simulink model "main_model"  (R2018b)
settings: Solver=VariableStepAuto  StartTime=0.0  StopTime=25  RelTol=1e-1
values from neighbouring files (symbols this model uses):
  beq = bm + bl/r^2    (= 1.5e-05)    [data.m]
  Cts = 1.091    [data.m]
  Jeq = Jm + Jl/r^2    (= 0.25041)    [data.m]
  lambda_rm = 0.01546    [data.m]
  Ld = 0.27e-3    (= 0.00027)    [data.m]
  Lls = 0.07e-3    (= 7e-05)    [data.m]
  Lq = 0.2e-3    (= 0.0002)    [data.m]
  Pp = 15    [data.m]
  r = 1    [data.m]
  Rs = 0.13    [data.m]
  Rts_amb = 55    [data.m]
  Tamb_max = 40    [data.m]
undefined symbols (not defined in the file or in its folder): ba, ke_omega, ke_theta, kei, ksa, ksia, R0p, Rdp, Rqp, sigbuilder_block
settings Model: Creator=Acer  LastModifiedBy=admin

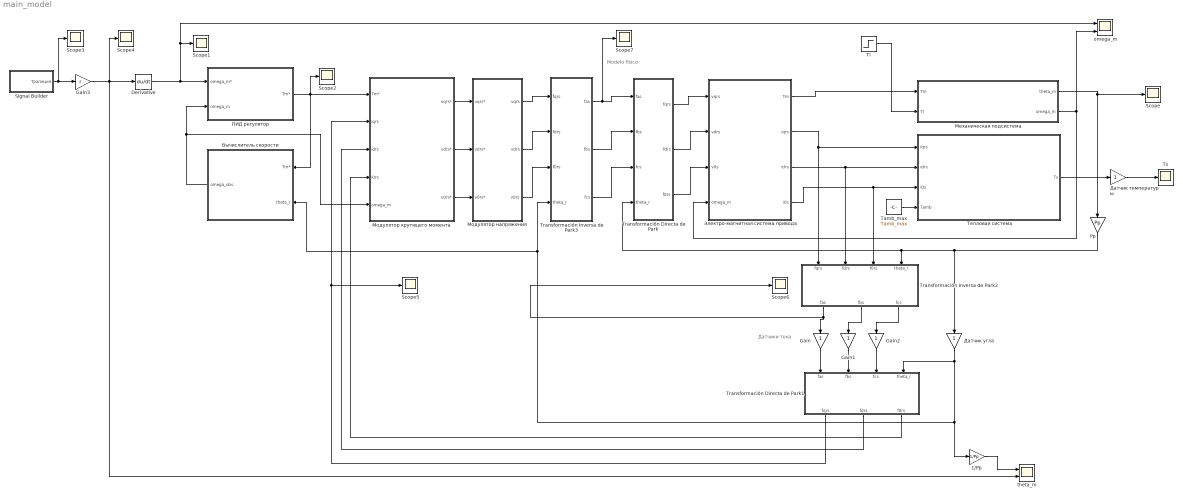
== system main_model ==
  note: Датчики тока
  note: Modelo físico
  " Датчик угла" : Gain
  1/Pp : Gain  Gain=1/Pp
  Derivative : Derivative  CoefficientInTFapproximation=Inf
  Gain : Gain
  Gain1 : Gain
  Gain2 : Gain
  Gain3 : Gain  Gain=r
  Pp : Gain  Gain=Pp
  Scope{,1..7} (8 alike) : Scope
  Signal Builder : Subsystem  Tag=STV Subsys  LoadFcn=sigbuilder_block('load');  StartFcn=sigbuilder_block('start');  StopFcn=sigbuilder_block('stop');  ClipboardFcn=sigbuilder_block('clipboard');  mask(Sigbuilder block){tuvar=[0:10]}
      mask help: Simulink:masks:SigbuilderBlock_MD
      mask init:
      | if ~strcmp(get_param(bdroot(gcbh),'SimulationStatus'),'stopped') tuvar = sigbuilder_block('maskInit'); end
      settings: CopyFcn=sigbuilder_block('copy');  DeleteFcn=sigbuilder_block('delete');  ModelCloseFcn=sigbuilder_block('modelClose');  PreSaveFcn=sigbuilder_block('preSave');  PauseFcn=sigbuilder_block('pause');  ContinueFcn=sigbuilder_block('continue');  NameChangeFcn=sigbuilder_block('namechange');  OpenFcn=sigbuilder_block('open',[113.25 126.75 960 498.75 ]);  CloseFcn=sigbuilder_block('close');
      mask Display: plot(0, 0, 100, 100,[2, 2, 32, 32, 2], [68, 8, 8, 68, 68],[32, 2], [38, 38], [32, 19, 2],[53, 60, 44], [32, 17, 17, 2],[16, 16, 31, 31]);txt = getActiveGroup(gcbh);text(2, 100, txt,'verticalAlignment', 'top');
  Tamb_max : Constant  Value=Tamb_max
  Tl : Step  Time=0.3  After=5.2  SampleTime=0
  Transformación Directa de Park : MATLAB Function  TreatAsAtomicUnit=on
  Transformación Directa de Park1 : MATLAB Function  TreatAsAtomicUnit=on
  Transformación Inversa de Park2 : MATLAB Function  TreatAsAtomicUnit=on
  Transformación Inversa de Park3 : MATLAB Function  TreatAsAtomicUnit=on
  Ts : Scope
  omega_m : Scope  NumInputPorts=2
  theta_m : Scope  NumInputPorts=2
  Вычислитель скорости : Subsystem
  Датчик температуры : Gain
  Механическая подсистема : Subsystem
  Модулятор крутящего момента : Subsystem
  Модулятор напряжения : Subsystem
  ПИД регулятор : Subsystem
  Тепловая система : Subsystem
  Электро-магнитная система привода : Subsystem
  wires:
  Механическая подсистема/1(theta_m) -> Scope/1, Pp/1
  Механическая подсистема/2(omega_m) -> omega_m/2, Электро-магнитная система привода/4(omega_m)
  Электро-магнитная система привода/2(iqrs) -> Transformación Inversa de Park2/1(fqrs), Тепловая система/1(iqrs)
  Электро-магнитная система привода/1(Tm) -> Механическая подсистема/1(Tm)
  Электро-магнитная система привода/4(i0s) -> Тепловая система/3(i0s), Transformación Inversa de Park2/3(f0rs)
  Тепловая система/1(Ts) -> Датчик температуры/1
  Tamb_max/1 -> Тепловая система/4(Tamb)
  Pp/1 -> " Датчик угла"/1, Transformación Directa de Park/4(theta_r), Transformación Inversa de Park2/4(theta_r)
  Электро-магнитная система привода/3(idrs) -> Тепловая система/2(idrs), Transformación Inversa de Park2/2(fdrs)
  Модулятор напряжения/1(vqrs) -> Transformación Inversa de Park3/1(fqrs)
  Модулятор напряжения/2(vdrs) -> Transformación Inversa de Park3/2(fdrs)
  Модулятор напряжения/3(v0rs) -> Transformación Inversa de Park3/3(f0rs)
  ПИД регулятор/1(Tm*) -> Scope2/1, Вычислитель скорости/1(Tm*), Модулятор крутящего момента/1(Tm*)
  Transformación Directa de Park1/3(f0rs) -> Модулятор крутящего момента/4(i0rs)
  Модулятор крутящего момента/1(vqrs*) -> Модулятор напряжения/1(vqrs*)
  Модулятор крутящего момента/2(vdrs*) -> Модулятор напряжения/2(vdrs*)
  Модулятор крутящего момента/3(v0rs*) -> Модулятор напряжения/3(v0rs*)
  Transformación Inversa de Park3/2(fbs) -> Transformación Directa de Park/2(fbs)
  Transformación Inversa de Park3/3(fcs) -> Transformación Directa de Park/3(fcs)
  Transformación Directa de Park/1(fqrs) -> Электро-магнитная система привода/1(vqrs)
  Transformación Directa de Park/2(fdrs) -> Электро-магнитная система привода/2(vdrs)
  Transformación Directa de Park/3(f0rs) -> Электро-магнитная система привода/3(v0s)
  Tl/1 -> Механическая подсистема/2(Tl)
  " Датчик угла"/1 -> Вычислитель скорости/2(theta_r), Transformación Inversa de Park3/4(theta_r), 1/Pp/1, Transformación Directa de Park1/4(theta_r)
  Transformación Inversa de Park2/3(fcs) -> Gain2/1
  Transformación Inversa de Park2/2(fbs) -> Gain1/1
  Transformación Inversa de Park2/1(fas) -> Scope6/1, Gain/1
  Transformación Directa de Park1/2(fdrs) -> Модулятор крутящего момента/3(idrs)
  Transformación Directa de Park1/1(fqrs) -> Scope5/1, Модулятор крутящего момента/2(iqrs)
  Датчик температуры/1 -> Ts/1
  Gain2/1 -> Transformación Directa de Park1/3(fcs)
  Gain1/1 -> Transformación Directa de Park1/2(fbs)
  Gain/1 -> Transformación Directa de Park1/1(fas)
  Вычислитель скорости/1(omega_obs) -> ПИД регулятор/2(omega_m), Модулятор крутящего момента/5(omega_m)
  Derivative/1 -> Scope1/1, omega_m/1, ПИД регулятор/1(omega_m*)
  Gain3/1 -> theta_m/2, Scope4/1, Derivative/1
  1/Pp/1 -> theta_m/1
  Signal Builder/1(Трапеция) -> Scope3/1, Gain3/1
  Transformación Inversa de Park3/1(fas) -> Scope7/1, Transformación Directa de Park/1(fas)

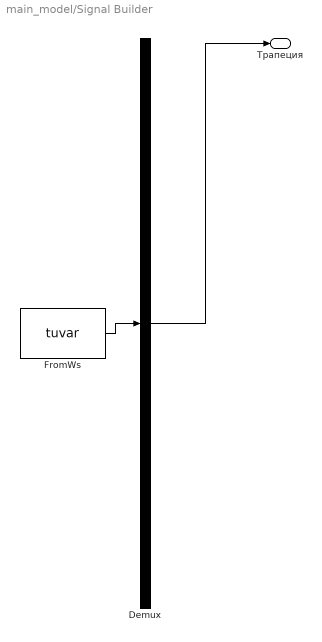
== system main_model/Signal Builder ==
  Demux : Demux  Tag=STV Demux  Outputs=1
  FromWs : FromWorkspace  Tag=STV FromWs  VariableName=tuvar  SampleTime=0
      SigBuilderData=|
      | common.afterFinalStr = 'Extrapolate'
      | common.sampleTime = 0
      | dataSet.timeRange = [0 30]
      | dataSet.name = 'Group 1'
      | sbobj.Groups.Name = 'Group 1'
      | sbobj.Groups.Signals.Name = 'Трапеция'
      | sbobj.Groups.Signals.XData = [0 5 8 14 17 30]
      | sbobj.Groups.Signals.YData = [0 0 30 30 0 0]
      | sbobj.Groups.TimeRange = [0 30]
  Трапеция : Outport  Tag=STV Outport
  wires:
  Demux/1 -> Трапеция/1
  FromWs/1 -> Demux/1

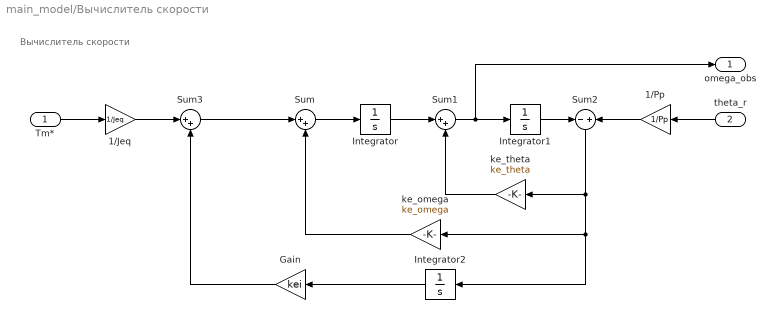
== system main_model/Вычислитель скорости ==
  note: Вычислитель скорости
  Tm* : Inport
  theta_r : Inport  Port=2
  1/Jeq : Gain  Gain=1/Jeq
  1/Pp : Gain  Gain=1/Pp
  Gain : Gain  Gain=kei
  Integrator : Integrator
  Integrator1 : Integrator
  Integrator2 : Integrator
  Sum : Sum  Inputs=|++
  Sum1 : Sum  Inputs=|++
  Sum2 : Sum  Inputs=-|+
  Sum3 : Sum  Inputs=|++
  ke_omega : Gain  Gain=ke_omega
  ke_theta : Gain  Gain=ke_theta
  omega_obs : Outport
  wires:
  Sum2/1 -> ke_theta/1, Integrator2/1, ke_omega/1
  ke_omega/1 -> Sum/2
  Tm*/1 -> 1/Jeq/1
  Integrator/1 -> Sum1/1
  Sum/1 -> Integrator/1
  Sum1/1 -> omega_obs/1, Integrator1/1
  Integrator1/1 -> Sum2/1
  ke_theta/1 -> Sum1/2
  1/Pp/1 -> Sum2/2
  theta_r/1 -> 1/Pp/1
  1/Jeq/1 -> Sum3/1
  Sum3/1 -> Sum/1
  Integrator2/1 -> Gain/1
  Gain/1 -> Sum3/2

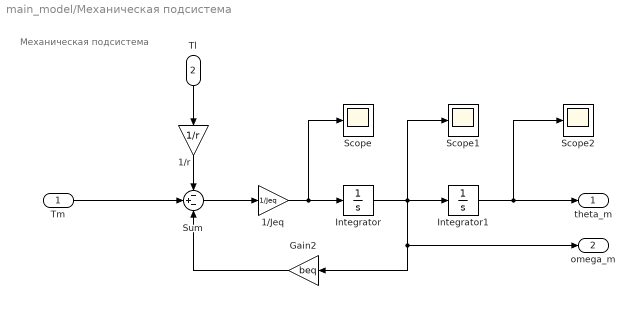
== system main_model/Механическая подсистема ==
  note: Механическая подсистема
  Tm : Inport
  Tl : Inport  Port=2
  1/Jeq : Gain  Gain=1/Jeq
  1/r : Gain  Gain=1/r
  Gain2 : Gain  Gain=beq
  Integrator : Integrator
  Integrator1 : Integrator
  Scope : Scope
  Scope1 : Scope
  Scope2 : Scope
  Sum : Sum  Inputs=-+-
  theta_m : Outport
  omega_m : Outport  Port=2
  wires:
  Integrator1/1 -> Scope2/1, theta_m/1
  Integrator/1 -> Scope1/1, omega_m/1, Gain2/1, Integrator1/1
  Tm/1 -> Sum/2
  1/r/1 -> Sum/1
  Sum/1 -> 1/Jeq/1
  Tl/1 -> 1/r/1
  Gain2/1 -> Sum/3
  1/Jeq/1 -> Scope/1, Integrator/1

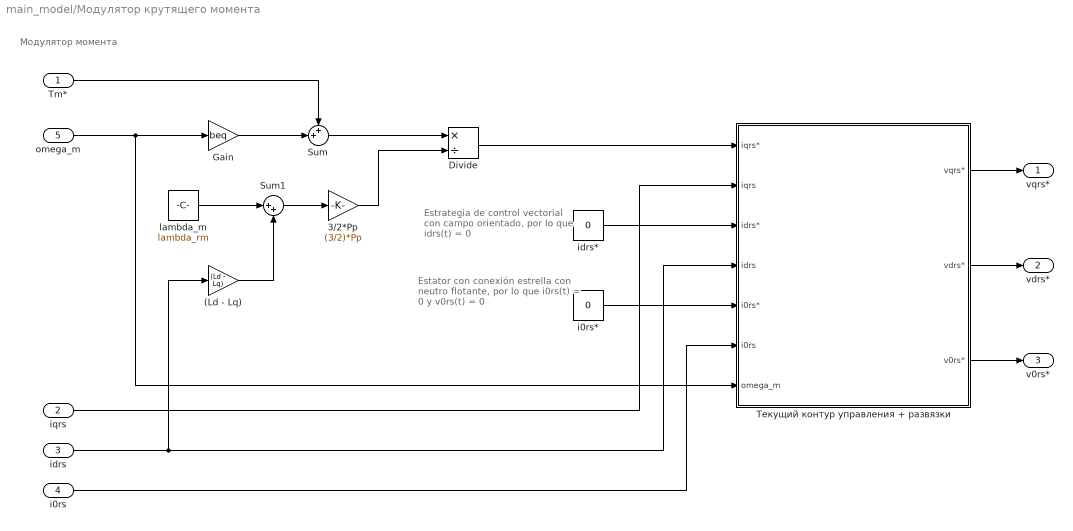
== system main_model/Модулятор крутящего момента ==
  note: Модулятор момента
  note: Estator con conexión estrella
      | con neutro flotante,
      | por lo que i0rs(t) = 0 y v0rs(t) = 0
  note: Estrategia de control vectorial
      | con campo orientado,
      | por lo que idrs(t) = 0
  Tm* : Inport
  iqrs : Inport  Port=2
  idrs : Inport  Port=3
  i0rs : Inport  Port=4
  omega_m : Inport  Port=5
  (Ld - Lq) : Gain  Gain=(Ld - Lq)
  3/2*Pp : Gain  Gain=(3/2)*Pp
  Divide : Product  Inputs=*/
  Gain : Gain  Gain=beq
  Sum : Sum  Inputs=++|
  Sum1 : Sum  Inputs=|++
  i0rs* : Constant  Value=0
  idrs* : Constant  Value=0
  lambda_m : Constant  Value=lambda_rm
  Текущий контур управления + развязки : Subsystem
  vqrs* : Outport
  vdrs* : Outport  Port=2
  v0rs* : Outport  Port=3
  wires:
  omega_m/1 -> Gain/1, Текущий контур управления + развязки/7(omega_m)
  i0rs*/1 -> Текущий контур управления + развязки/5(i0rs*)
  3/2*Pp/1 -> Divide/2
  (Ld - Lq)/1 -> Sum1/2
  Sum1/1 -> 3/2*Pp/1
  Divide/1 -> Текущий контур управления + развязки/1(iqrs*)
  Gain/1 -> Sum/2
  idrs*/1 -> Текущий контур управления + развязки/3(idrs*)
  Sum/1 -> Divide/1
  idrs/1 -> (Ld - Lq)/1, Текущий контур управления + развязки/4(idrs)
  i0rs/1 -> Текущий контур управления + развязки/6(i0rs)
  iqrs/1 -> Текущий контур управления + развязки/2(iqrs)
  lambda_m/1 -> Sum1/1
  Tm*/1 -> Sum/1
  Текущий контур управления + развязки/1(vqrs*) -> vqrs*/1
  Текущий контур управления + развязки/3(v0rs*) -> v0rs*/1
  Текущий контур управления + развязки/2(vdrs*) -> vdrs*/1

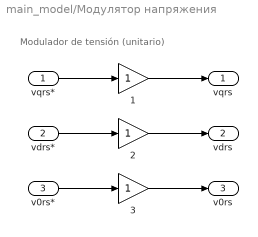
== system main_model/Модулятор напряжения ==
  note: Modulador de tensión (unitario)
  vqrs* : Inport
  vdrs* : Inport  Port=2
  v0rs* : Inport  Port=3
  1 : Gain
  2 : Gain
  3 : Gain
  vqrs : Outport
  vdrs : Outport  Port=2
  v0rs : Outport  Port=3
  wires:
  vqrs*/1 -> 1/1
  vdrs*/1 -> 2/1
  1/1 -> vqrs/1
  v0rs*/1 -> 3/1
  2/1 -> vdrs/1
  3/1 -> v0rs/1

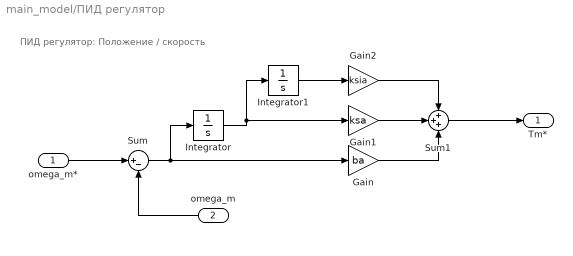
== system main_model/ПИД регулятор ==
  note: ПИД регулятор: Положение / скорость
  omega_m* : Inport
  omega_m : Inport  Port=2
  Gain : Gain  Gain=ba
  Gain1 : Gain  Gain=ksa
  Gain2 : Gain  Gain=ksia
  Integrator : Integrator
  Integrator1 : Integrator
  Sum : Sum  Inputs=|+-
  Sum1 : Sum  Inputs=+++
  Tm* : Outport
  wires:
  Integrator/1 -> Integrator1/1, Gain1/1
  Sum/1 -> Gain/1, Integrator/1
  Gain1/1 -> Sum1/2
  Gain/1 -> Sum1/3
  Integrator1/1 -> Gain2/1
  Gain2/1 -> Sum1/1
  omega_m/1 -> Sum/2
  Sum1/1 -> Tm*/1
  omega_m*/1 -> Sum/1

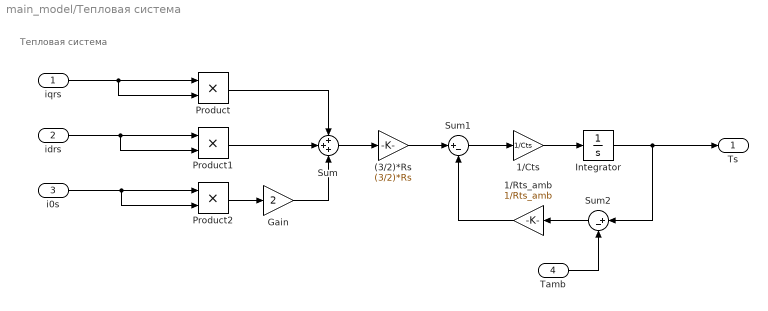
== system main_model/Тепловая система ==
  note: Тепловая система
  iqrs : Inport
  idrs : Inport  Port=2
  i0s : Inport  Port=3
  Tamb : Inport  Port=4
  (3/2)*Rs : Gain  Gain=(3/2)*Rs
  1/Cts : Gain  Gain=1/Cts
  1/Rts_amb : Gain  Gain=1/Rts_amb
  Gain : Gain  Gain=2
  Integrator : Integrator  InitialCondition=Tamb_max
  Product : Product
  Product1 : Product
  Product2 : Product
  Sum : Sum  Inputs=+++
  Sum1 : Sum  Inputs=|+-
  Sum2 : Sum  Inputs=|+-
  Ts : Outport
  wires:
  Integrator/1 -> Ts/1, Sum2/1
  1/Cts/1 -> Integrator/1
  i0s/1 -> Product2/2, Product2/1
  Product/1 -> Sum/1
  Sum2/1 -> 1/Rts_amb/1
  (3/2)*Rs/1 -> Sum1/1
  Tamb/1 -> Sum2/2
  Sum/1 -> (3/2)*Rs/1
  1/Rts_amb/1 -> Sum1/2
  Gain/1 -> Sum/3
  Sum1/1 -> 1/Cts/1
  iqrs/1 -> Product/2, Product/1
  idrs/1 -> Product1/2, Product1/1
  Product2/1 -> Gain/1
  Product1/1 -> Sum/2

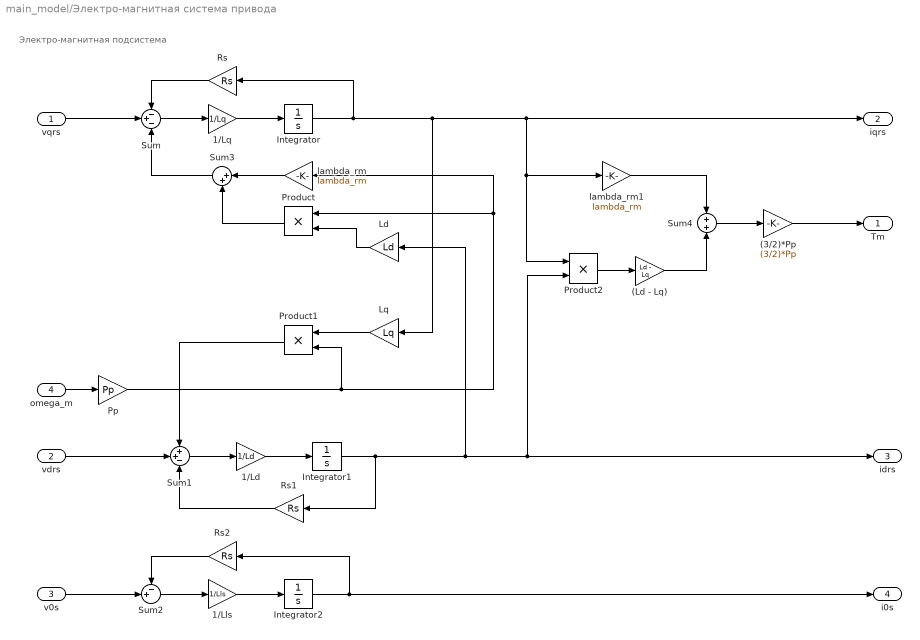
== system main_model/Электро-магнитная система привода ==
  note: Электро-магнитная подсистема
  vqrs : Inport
  vdrs : Inport  Port=2
  v0s : Inport  Port=3
  omega_m : Inport  Port=4
  (3/2)*Pp : Gain  Gain=(3/2)*Pp
  (Ld - Lq) : Gain  Gain=Ld - Lq
  1/Ld : Gain  Gain=1/Ld
  1/Lls : Gain  Gain=1/Lls
  1/Lq : Gain  Gain=1/Lq
  Integrator : Integrator
  Integrator1 : Integrator
  Integrator2 : Integrator
  Ld : Gain  Gain=Ld
  Lq : Gain  Gain=Lq
  Pp : Gain  Gain=Pp
  Product : Product
  Product1 : Product
  Product2 : Product
  Rs : Gain  Gain=Rs
  Rs1 : Gain  Gain=Rs
  Rs2 : Gain  Gain=Rs
  Sum : Sum  Inputs=-+-
  Sum1 : Sum  Inputs=++-
  Sum2 : Sum  Inputs=-+|
  Sum3 : Sum  Inputs=|++
  Sum4 : Sum  Inputs=+|+
  lambda_rm : Gain  Gain=lambda_rm
  lambda_rm1 : Gain  Gain=lambda_rm
  Tm : Outport
  iqrs : Outport  Port=2
  idrs : Outport  Port=3
  i0s : Outport  Port=4
  wires:
  lambda_rm/1 -> Sum3/1
  Product1/1 -> Sum1/1
  Lq/1 -> Product1/1
  Pp/1 -> lambda_rm/1, Product/1, Product1/2
  Product/1 -> Sum3/2
  vdrs/1 -> Sum1/2
  1/Lq/1 -> Integrator/1
  vqrs/1 -> Sum/2
  omega_m/1 -> Pp/1
  Integrator1/1 -> Ld/1, Product2/2, idrs/1, Rs1/1
  Sum1/1 -> 1/Ld/1
  Integrator/1 -> Rs/1, Lq/1, iqrs/1, Product2/1, lambda_rm1/1
  Sum2/1 -> 1/Lls/1
  Integrator2/1 -> i0s/1, Rs2/1
  Sum3/1 -> Sum/3
  Rs1/1 -> Sum1/3
  Sum4/1 -> (3/2)*Pp/1
  Ld/1 -> Product/2
  lambda_rm1/1 -> Sum4/1
  (3/2)*Pp/1 -> Tm/1
  1/Ld/1 -> Integrator1/1
  Rs2/1 -> Sum2/1
  Rs/1 -> Sum/1
  Product2/1 -> (Ld - Lq)/1
  (Ld - Lq)/1 -> Sum4/2
  Sum/1 -> 1/Lq/1
  1/Lls/1 -> Integrator2/1
  v0s/1 -> Sum2/2

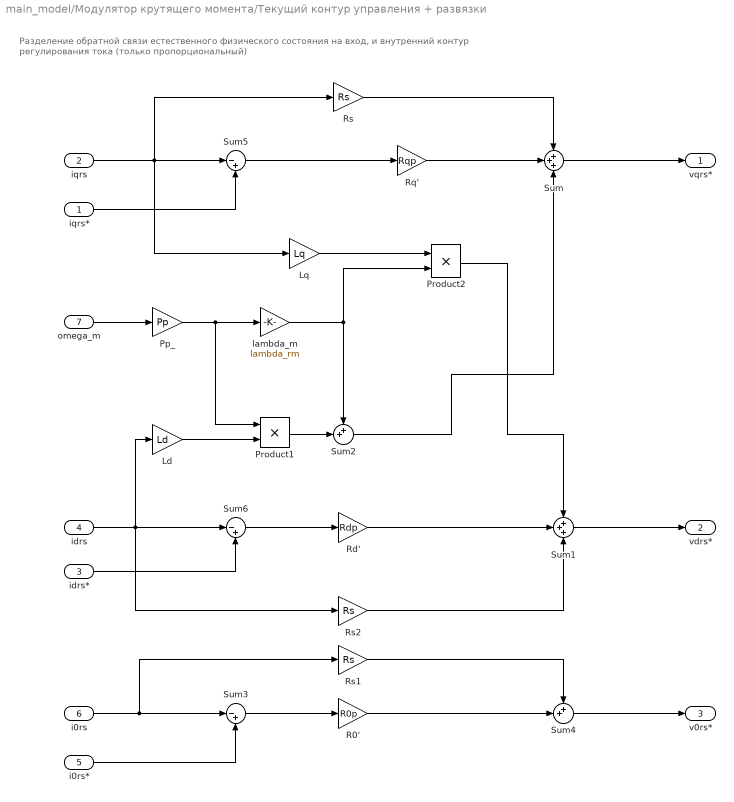
== system main_model/Модулятор крутящего момента/Текущий контур управления + развязки ==
  note: Разделение обратной связи естественного физического состояния на вход,
      | и внутренний контур регулирования тока (только пропорциональный)
  iqrs* : Inport
  iqrs : Inport  Port=2
  idrs* : Inport  Port=3
  idrs : Inport  Port=4
  i0rs* : Inport  Port=5
  i0rs : Inport  Port=6
  omega_m : Inport  Port=7
  Ld : Gain  Gain=Ld
  Lq : Gain  Gain=Lq
  Pp_ : Gain  Gain=Pp
  Product1 : Product
  Product2 : Product
  R0' : Gain  Gain=R0p
  Rd' : Gain  Gain=Rdp
  Rq' : Gain  Gain=Rqp
  Rs : Gain  Gain=Rs
  Rs1 : Gain  Gain=Rs
  Rs2 : Gain  Gain=Rs
  Sum : Sum  Inputs=+++
  Sum1 : Sum  Inputs=+++
  Sum2 : Sum  Inputs=++|
  Sum3 : Sum  Inputs=|-+
  Sum4 : Sum  Inputs=++|
  Sum5 : Sum  Inputs=|-+
  Sum6 : Sum  Inputs=|-+
  lambda_m : Gain  Gain=lambda_rm
  vqrs* : Outport
  vdrs* : Outport  Port=2
  v0rs* : Outport  Port=3
  wires:
  omega_m/1 -> Pp_/1
  lambda_m/1 -> Product2/2, Sum2/1
  i0rs*/1 -> Sum3/2
  Pp_/1 -> Product1/1, lambda_m/1
  Rq'/1 -> Sum/2
  R0'/1 -> Sum4/2
  i0rs/1 -> Sum3/1, Rs1/1
  Sum3/1 -> R0'/1
  Sum4/1 -> v0rs*/1
  Sum1/1 -> vdrs*/1
  Product2/1 -> Sum1/1
  idrs*/1 -> Sum6/2
  Sum/1 -> vqrs*/1
  Sum6/1 -> Rd'/1
  idrs/1 -> Ld/1, Rs2/1, Sum6/1
  Sum5/1 -> Rq'/1
  iqrs/1 -> Lq/1, Sum5/1, Rs/1
  Lq/1 -> Product2/1
  Sum2/1 -> Sum/3
  Rs2/1 -> Sum1/3
  Rs1/1 -> Sum4/1
  Rs/1 -> Sum/1
  Rd'/1 -> Sum1/2
  Ld/1 -> Product1/2
  iqrs*/1 -> Sum5/2
  Product1/1 -> Sum2/2

== matlab function main_model/Transformación Inversa de Park2 ==
  data: fqrs input; fdrs input; f0rs input; theta_r input; fas output; fbs output; fcs output
function [fas, fbs, fcs] = dq0_inverse( fqrs, fdrs, f0rs, theta_r )
% ОБРАТНОЕ ПРЕОБРАЗОВАНИЕ ПАРКА 
%   Прямое преобразование для перехода от трехфазных координат 
%   от статора abc до фиксированных координат ротора qd0.
fqd0 = [ fqrs; fdrs; f0rs ];

A = [ 
    cos(theta_r)            sin(theta_r)            1;
    cos(theta_r - 2*pi/3)   sin(theta_r - 2*pi/3)   1;
    cos(theta_r + 2*pi/3)   sin(theta_r + 2*pi/3)   1
    ];

fabc =  A * fqd0;

fas = fabc(1);
fbs = fabc(2);
fcs = fabc(3);

end

== matlab function main_model/Transformación Directa de Park ==
  data: fas input; fbs input; fcs input; theta_r input; fqrs output; fdrs output; f0rs output
function [fqrs, fdrs, f0rs] = dq0_direct( fas, fbs, fcs, theta_r )
% ПРЯМОЕ ПРЕОБРАЗОВАНИЕ ПАРКА 
%   Прямое преобразование для перехода от трехфазных координат 
%   статора abc относительно фиксированных координат ротора qd0. 
fabc = [ fas; fbs; fcs ];

A = [ 
    cos(theta_r)    cos(theta_r - 2*pi/3)   cos(theta_r + 2*pi/3);
    sin(theta_r)    sin(theta_r - 2*pi/3)   sin(theta_r + 2*pi/3);
    0.5             0.5                     0.5
    ];

fqd0 = (2/3) * A * fabc;

fqrs = fqd0(1);
fdrs = fqd0(2);
f0rs = fqd0(3);

end

== matlab function main_model/Transformación Directa de Park1 ==
  data: fas input; fbs input; fcs input; theta_r input; fqrs output; fdrs output; f0rs output
function [fqrs, fdrs, f0rs] = dq0_direct( fas, fbs, fcs, theta_r )
% ПРЯМОЕ ПРЕОБРАЗОВАНИЕ ПАРКА 
%   Прямое преобразование для перехода от трехфазных координат 
%   от статора abc до фиксированных координат ротора qd0.
fabc = [ fas; fbs; fcs ];

A = [ 
    cos(theta_r)    cos(theta_r - 2*pi/3)   cos(theta_r + 2*pi/3);
    sin(theta_r)    sin(theta_r - 2*pi/3)   sin(theta_r + 2*pi/3);
    0.5             0.5                     0.5
    ];

fqd0 = (2/3) * A * fabc;

fqrs = fqd0(1);
fdrs = fqd0(2);
f0rs = fqd0(3);

end

== matlab function main_model/Transformación Inversa de Park3 ==
  data: fqrs input; fdrs input; f0rs input; theta_r input; fas output; fbs output; fcs output
function [fas, fbs, fcs] = dq0_inverse( fqrs, fdrs, f0rs, theta_r )
% ОБРАТНОЕ ПРЕОБРАЗОВАНИЕ ПАРКА 
%   Прямое преобразование для перехода от трехфазных координат 
%   от статора abc до фиксированных координат ротора qd0
fqd0 = [ fqrs; fdrs; f0rs ];

A = [ 
    cos(theta_r)            sin(theta_r)            1;
    cos(theta_r - 2*pi/3)   sin(theta_r - 2*pi/3)   1;
    cos(theta_r + 2*pi/3)   sin(theta_r + 2*pi/3)   1
    ];

fabc =  A * fqd0;

fas = fabc(1);
fbs = fabc(2);
fcs = fabc(3);

end
